simulink model "ACMotorSkalarControl"  (R2019a)
settings: Solver=VariableStepAuto  StartTime=0.0  StopTime=5  RelTol=1e-3
libraries: powerlib x10, simulink x3, powerlib_meascontrol x1
settings Model: Creator=90538  LastModifiedBy=Furkan

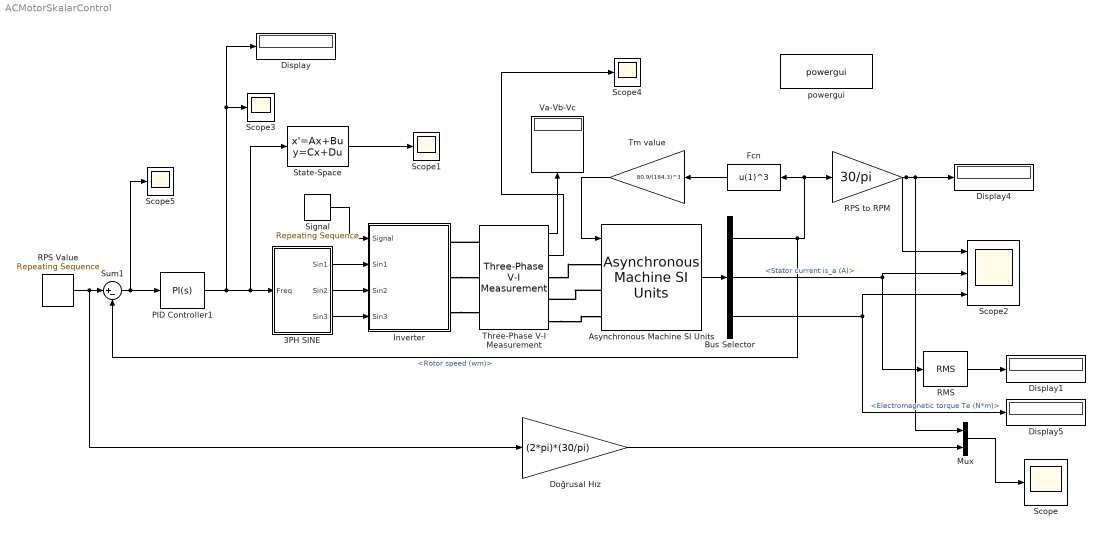
== system ACMotorSkalarControl ==
  " Inverter" : Subsystem
  3PH SINE : Subsystem
  Asynchronous Machine SI Units : powerlib/Machines/Asynchronous Machine SI Units  RotorType=Squirrel-cage  PresetModel="03:  20 HP  460 V 60Hz 1760 RPM"  MechanicalLoad=Torque Tm  ShowDetailedParameters=on  ReferenceFrame=Rotor  Units=SI  MeasurementBus=off  NominalParameters=[1.492e+04 460 60]  Stator=[0.2761 0.002191]  Rotor=[0.1645 0.002191]  Cage1=[0.4155 0.002066]  Cage2=[0.4168 0.0003495]  Lm=0.07614  Mechanical=[0.1 0.01771 2]  PolePairs=2  InitialConditions=[1 0 0 0 0 0 0 0]  SimulateSaturation=off  Saturation=[14.03593122, 27.81365428, 53.79336849, 72.68890987, 97.98006896, 148.6815601, 215.7428561, 302.9841135, 428.7778367 ; 230, 322, 414, 460, 506, 552, 598, 644, 690]  LoadFlowParameters=1492000  TsPowergui=0  TsBlock=-1  IterativeModel=Trapezoidal non iterative  IterativeDiscreteModel=Trapezoidal non iterative  Pmec=1.492e+006
      settings: SourceProductName=Simscape Electrical
  Bus Selector : BusSelector  OutputSignals=Mechanical.Rotor speed (wm),Stator measurements.Stator current is_a (A),Mechanical.Electromagnetic torque Te (N*m)
  Display{,1,4..5} (4 alike) : Display
  "Doğrusal Hız " : Gain  Gain=(2*pi)*(30/pi)
  Fcn : Fcn  Expr=u(1)^3
  Mux : Mux  Inputs=2
  PID Controller1 : simulink/Continuous/PID Controller  Controller=PI  Form=Parallel  TimeDomain=Continuous-time  SampleTime=-1  IntegratorMethod=Forward Euler  FilterMethod=Forward Euler  ControllerParametersSource=internal  P=0.02  I=1  D=0.05  UseFilter=on  N=100  TunerSelectOption=Transfer Function Based (PID Tuner App)  InitialConditionSource=internal  InitialConditionForIntegrator=0  InitialConditionForFilter=0  DifferentiatorICPrevScaledInput=0  ExternalReset=none  TrackingMode=off  Kt=1  LimitOutput=on  UpperSaturationLimit=60  LowerSaturationLimit=-60  LinearizeAsGain=on  AntiWindupMode=clamping  Kb=1  POutMin=[]  POutMax=[]  IOutMin=[]  IOutMax=[]  DOutMin=[]  DOutMax=[]  NOutMin=[]  NOutMax=[]  SumOutMin=[]  SumOutMax=[]  SaturationOutMin=[]  SaturationOutMax=[]  PParamMin=[]  PParamMax=[]  IParamMin=[]  IParamMax=[]  DParamMin=[]  DParamMax=[]  NParamMin=[]  NParamMax=[]  KbParamMin=[]  KbParamMax=[]  KtParamMin=[]  KtParamMax=[]  KbOutMin=[]  KbOutMax=[]  KtOutMin=[]  KtOutMax=[]  IntegratorOutMin=[]  IntegratorOutMax=[]  FilterOutMin=[]  FilterOutMax=[]  SumI1OutMin=[]  SumI1OutMax=[]  SumI2OutMin=[]  SumI2OutMax=[]  SumI3OutMin=[]  SumI3OutMax=[]  SumI4OutMin=[]  SumI4OutMax=[]  SumDOutMin=[]  SumDOutMax=[]  DifferentiatorOutMin=[]  DifferentiatorOutMax=[]  FilterDiffOutCoefMin=[]  FilterDiffOutCoefMax=[]  ReciprocalOutMin=[]  ReciprocalOutMax=[]  SumDenOutMin=[]  SumDenOutMax=[]  SumNumOutMin=[]  SumNumOutMax=[]  DivideOutMin=[]  DivideOutMax=[]  IntegratorContinuousStateAttributes=''  IntegratorStateMustResolveToSignalObject=off  IntegratorRTWStateStorageClass=Auto  FilterContinuousStateAttributes=''  FilterStateMustResolveToSignalObject=off  FilterRTWStateStorageClass=Auto  ParallelPVariant=InternalParameters  IdealPVariant=Disabled  IVariant=InternalParameters  DVariant=Disabled  IntegratorVariant=Continuous  SatVariant=Enabled  AWVariant=ContClampingParallel  PCopyVariant=Disabled  TRVariant=Disabled  FdbkBlocksVariant=Forward  IdealPFdbkVariant=Disabled  SatFdbkVariant=Disabled  DerivativeFilterVariant=Disabled  NVariant=Disabled  NCopyVariant=Disabled_SignalSpec  FilterICVariant=Disabled  IntegratorICVariant=InternalICs  ExternalResetVariant=Disabled  TRSumVariant=Passthrough  SumFdbkVariant=Disabled  SumVariant=Sum_PI
  RMS : powerlib_meascontrol/Measurements/RMS  TrueRMS=on  Freq=60  RMSInit=120  Ts=0
      settings: SourceProductName=Simscape Electrical
  RPS Value : simulink/Sources/Repeating Sequence  rep_seq_t=[0 .2 5]  rep_seq_y=[0 184 184]
  "RPS to RPM " : Gain  Gain=30/pi
  Scope{,1,3..5} (5 alike) : Scope
  Scope2 : Scope  NumInputPorts=3
  "Signal " : simulink/Sources/Repeating Sequence  rep_seq_t=[0 0.25 0.50 0.75 1]/2000  rep_seq_y=[0 1 0 -1 0]
  State-Space : StateSpace  A=[-63.9015 -71.4367 0; -62.1141 -73.4924 0; -1.7874 2.0557 0]  B=|  C=[0 1 0]  D=[0]  InitialCondition=0
      | [ -443.2787
      | ;  456.4128
      | ;   13.1339
      | ]
  Sum1 : Sum  Inputs=|+-
  Three-Phase V-I Measurement : powerlib/Measurements/Three-Phase V-I Measurement  VoltageMeasurement=phase-to-phase  SetLabelV=off  LabelV=Vabc  Vpu=off  VpuLL=off  CurrentMeasurement=yes  SetLabelI=off  LabelI=Iabc  Ipu=off  Pbase=100e6  Vbase=500e3  OutputType=Complex  PhasorSimulation=off  PSBequivalent=0
      settings: SourceProductName=Simscape Electrical
  Tm value : Gain  Gain=80.9/(184.3)^3
  Va-Vb-Vc : Display
  powergui : powerlib/powergui  Priority=1  SimulationMode=Discrete  SampleTime=1e-6  frequency=60  Iterations=50  frequencyindice=60  Pbase=100e6  ErrMax=1e-4  UnitsV=kV  UnitsW=MW  buscounter=0  FunctionMessages=off  echomessages=off  EnableUseOfTLC=off  CurrentSourceSwitches=off  DisableSnubberDevices=off  DisableRonSwitches=off  DisableVfSwitches=off  DisplayEquations=off  AutomaticDiscreteSolvers=off  SolverType=Tustin/Backward Euler (TBE)  Interpol=off  ExternalGateDelay=off  methode=off  Ts=100  x0status=blocks  SPID=on  SwTol=0  HookPort=off  NonlinearTolerance=0  nMaxIteration=15  ContinueOnMaxIteration=off  RestoreLinks=warning  ResistiveCurrentMeasurement=off  Frange=[0:2:500]  Ylog=off  Xlog=on  ShowGrid=off  save=off  variable=ZData  structure=0  ZoomFFT=off  StartTime=0.0  cycles=1  DisplayStyle=1  fundamental=60  FreqAxis=off  MaxFrequency=1000  frequencyindicesteady=1  RmsSteady=1  display=off
      settings: SourceProductName=Simscape Electrical
  wires:
  Bus Selector/3 -> Scope2/3, Display5/1  "<Electromagnetic torque Te (N*m)>"
  Bus Selector/2 -> RMS/1, Scope2/2  "<Stator current is_a (A)>"
  "RPS to RPM "/1 -> Scope2/1, Mux/1, Display4/1
  RMS/1 -> Display1/1
  "Signal "/1 -> " Inverter"/1("Signal ")
  3PH SINE/3("Sin3 ") -> " Inverter"/4(Sin3)
  3PH SINE/2(Sin2) -> " Inverter"/3(Sin2)
  3PH SINE/1(Sin1) -> " Inverter"/2(Sin1)
  Three-Phase V-I Measurement/1 -> Va-Vb-Vc/1
  Fcn/1 -> Tm value/1
  Bus Selector/1 -> Fcn/1, "RPS to RPM "/1, Sum1/2  "<Rotor speed (wm)>"
  Tm value/1 -> Asynchronous Machine SI Units/1
  Asynchronous Machine SI Units/1 -> Bus Selector/1
  State-Space/1 -> Scope1/1
  Sum1/1 -> Scope5/1, PID Controller1/1
  PID Controller1/1 -> State-Space/1, 3PH SINE/1("Freq "), Display/1, Scope3/1
  RPS Value/1 -> "Doğrusal Hız "/1, Sum1/1
  "Doğrusal Hız "/1 -> Mux/2
  Mux/1 -> Scope/1
  Three-Phase V-I Measurement/2 -> Scope4/1
  connections:
  " Inverter"/RConn3 -- Three-Phase V-I Measurement/LConn3
  Three-Phase V-I Measurement/RConn3 -- Asynchronous Machine SI Units/LConn3
  Three-Phase V-I Measurement/LConn1 -- " Inverter"/RConn1
  Asynchronous Machine SI Units/LConn2 -- Three-Phase V-I Measurement/RConn2
  " Inverter"/RConn2 -- Three-Phase V-I Measurement/LConn2
  Three-Phase V-I Measurement/RConn1 -- Asynchronous Machine SI Units/LConn1

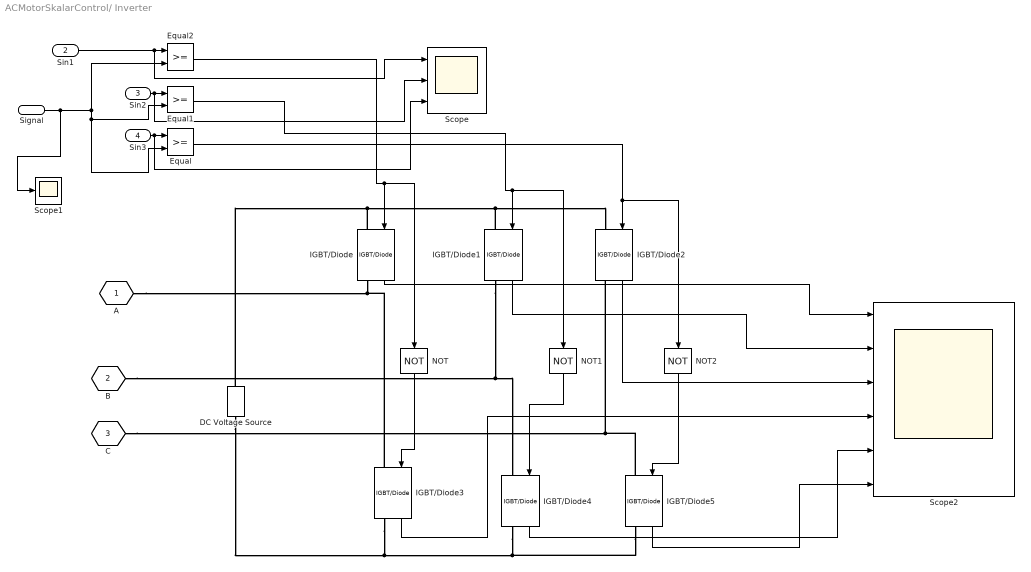
== system ACMotorSkalarControl/ Inverter ==
  "Signal " : Inport
  Sin1 : Inport  Port=2
  Sin2 : Inport  Port=3
  Sin3 : Inport  Port=4
  DC Voltage Source : powerlib/Electrical Sources/DC Voltage Source  Amplitude=600  Measurements=None
      settings: SourceProductName=Simscape Electrical
  Equal : RelationalOperator  OutDataTypeStr=boolean  RndMeth=Simplest
  Equal1 : RelationalOperator  OutDataTypeStr=boolean  RndMeth=Simplest
  Equal2 : RelationalOperator  OutDataTypeStr=boolean  RndMeth=Simplest
  IGBT/Diode{,1..5} (6 alike) : powerlib/Power Electronics/IGBT//Diode  Ron=1e-3  Rs=1e5  Cs=inf  Measurements=on
      settings: SourceProductName=Simscape Electrical
  NOT : Logic  Operator=NOT  IconShape=distinctive  AllPortsSameDT=off  OutDataTypeStr=boolean
  NOT1 : Logic  Operator=NOT  IconShape=distinctive  AllPortsSameDT=off  OutDataTypeStr=boolean
  NOT2 : Logic  Operator=NOT  IconShape=distinctive  AllPortsSameDT=off  OutDataTypeStr=boolean
  Scope : Scope  NumInputPorts=3
  Scope1 : Scope
  Scope2 : Scope  NumInputPorts=6
  "A " : PMIOPort  Tag=PMCPort  Side=Right
  "B " : PMIOPort  Tag=PMCPort  Port=2  Side=Right
  "C " : PMIOPort  Tag=PMCPort  Port=3  Side=Right
  wires:
  Sin3/1 -> Scope/3, Equal/1
  Sin1/1 -> Scope/1, Equal2/1
  Sin2/1 -> Scope/2, Equal1/1
  "Signal "/1 -> Scope1/1, Equal2/2, Equal/2, Equal1/2
  Equal2/1 -> NOT/1, IGBT/Diode/1
  Equal1/1 -> NOT1/1, IGBT/Diode1/1
  Equal/1 -> NOT2/1, IGBT/Diode2/1
  NOT/1 -> IGBT/Diode3/1
  NOT1/1 -> IGBT/Diode4/1
  NOT2/1 -> IGBT/Diode5/1
  IGBT/Diode2/1 -> Scope2/3
  IGBT/Diode1/1 -> Scope2/2
  IGBT/Diode/1 -> Scope2/1
  IGBT/Diode5/1 -> Scope2/6
  IGBT/Diode4/1 -> Scope2/5
  IGBT/Diode3/1 -> Scope2/4
  connections:
  DC Voltage Source/LConn1 -- IGBT/Diode3/RConn1 -- IGBT/Diode5/RConn1 -- IGBT/Diode4/RConn1
  DC Voltage Source/RConn1 -- IGBT/Diode/LConn1 -- IGBT/Diode1/LConn1 -- IGBT/Diode2/LConn1
  "C "/RConn1 -- IGBT/Diode5/LConn1 -- IGBT/Diode2/RConn1
  IGBT/Diode1/RConn1 -- "B "/RConn1 -- IGBT/Diode4/LConn1
  IGBT/Diode/RConn1 -- "A "/RConn1 -- IGBT/Diode3/LConn1

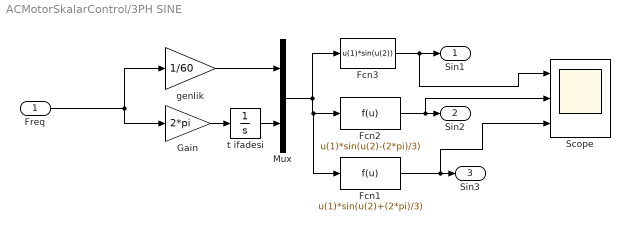
== system ACMotorSkalarControl/3PH SINE ==
  "Freq " : Inport
  Fcn1 : Fcn  Expr=u(1)*sin(u(2)+(2*pi)/3)
  Fcn2 : Fcn  Expr=u(1)*sin(u(2)-(2*pi)/3)
  Fcn3 : Fcn  Expr=u(1)*sin(u(2))
  Gain : Gain  Gain=2*pi
  Mux : Mux  Inputs=2
  Scope : Scope  NumInputPorts=3
  "genlik " : Gain  Gain=1/60
  "t ifadesi " : Integrator
  Sin1 : Outport
  Sin2 : Outport  Port=2
  "Sin3 " : Outport  Port=3
  wires:
  Gain/1 -> "t ifadesi "/1
  "genlik "/1 -> Mux/1
  "t ifadesi "/1 -> Mux/2
  Fcn1/1 -> Scope/3, "Sin3 "/1
  Mux/1 -> Fcn3/1, Fcn2/1, Fcn1/1
  "Freq "/1 -> Gain/1, "genlik "/1
  Fcn3/1 -> Scope/1, Sin1/1
  Fcn2/1 -> Scope/2, Sin2/1
